simulink model "projet_working"  (R2018a)
settings: Solver=FixedStepAuto  StartTime=0.0  StopTime=5  RelTol=1e-3  EnableMultiTasking=on
values from neighbouring files (symbols this model uses):
  a = [0 1 ; 0 -6.523]    [Project_state_space.m]
  b = [0;1]    [Project_state_space.m]
  c = [0.09667 0]    [Project_state_space.m]
  k = place(sysssD.a,sysssD.b,[0.9 0.7])    [Discret_LEGO_script.m]    (also in Project_state_space.m = place(a, b, P'); RLS_Glemselsfaktor.m = Q*Phi'; RLS_Kalman.m = Q*Phi'; RLS_Online.m = p*Phi')
  L_1 = [l_1; l_2]    [Project_state_space.m]
libraries: legoev3lib x2
settings Model: SimulationMode=external  ExtModeTrigDuration=2  Creator=Lenovo  LastModifiedBy=Lenovo
settings SolverCC: PositivePriorityOrder=on
settings OptimizationCC: EnhancedBackFolding=on  PassReuseOutputArgsThreshold=0  MaxStackSize=64  OptimizeBlockOrder=speed  DifferentSizesBufferReuse=on  OptimizationCustomize=off
settings DebuggingCC: ParameterTunabilityLossMsg=error
settings HardwareCC: ProdBitPerPointer=32  ProdBitPerSizeT=32  ProdBitPerPtrDiffT=32  ProdLargestAtomicInteger=Long  ProdWordSize=32  ProdHWDeviceType=ARM Compatible->ARM 9  UseEmbeddedCoderFeatures=off  UseSimulinkCoderFeatures=off
settings SFSimCC: MATLABDynamicMemAlloc=off
settings RTWCC: SystemTargetFile=ert.tlc  HardwareBoard=LEGO MINDSTORMS EV3  TLCOptions="-aInlineSetEventsForThisBaseRateFcn=TLC_FALSE -aSuppressMultiTaskScheduler=TLC_FALSE  -aRateBasedStepFcn=0"  TemplateMakefile=ert_default_tmf  GenerateReport=on  Toolchain=Sourcery G++ Lite v2009q3  LaunchReport=on
settings CodeAppCC: ForceParamTrailComments=on  OperatorAnnotations=on
settings ERTTargetCC: ERTCustomFileBanners=off  SupportContinuousTime=on  SupportNonInlinedSFcns=on  RemoveResetFunc=off  SupportVariableSizeSignals=on  ModelStepFunctionPrototypeControlCompliant=off

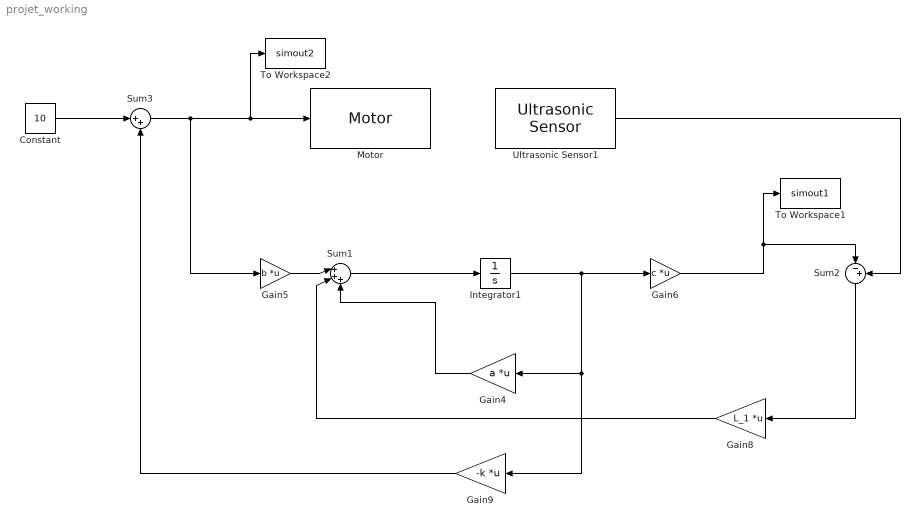
== system projet_working ==
  Constant : Constant  Value=10
  Gain4 : Gain  Gain=a  Multiplication=Matrix(K*u)
  Gain5 : Gain  Gain=b  Multiplication=Matrix(K*u)
  Gain6 : Gain  Gain=c  Multiplication=Matrix(K*u)
  Gain8 : Gain  Gain=L_1  Multiplication=Matrix(K*u)
  Gain9 : Gain  Gain=-k  Multiplication=Matrix(K*u)
  Integrator1 : Integrator
  Motor : legoev3lib/Motor  sportNumber=A  sstopAction=Brake
  Sum1 : Sum  Inputs=|+++
  Sum2 : Sum  Inputs=|-+
  Sum3 : Sum  Inputs=|++
  To Workspace1 : ToWorkspace  VariableName=simout1  SaveFormat=Structure With Time  SampleTime=-1
  To Workspace2 : ToWorkspace  VariableName=simout2  SaveFormat=Structure With Time  SampleTime=-1
  Ultrasonic Sensor1 : legoev3lib/Ultrasonic Sensor  PortNumber=1  sampleTime=0.1
      settings: SourceProductName=Simulink Support Package for LEGO MINDSTORMS EV3 Hardware  SourceProductBaseCode=LEGOEV3
  wires:
  Gain5/1 -> Sum1/1
  Gain9/1 -> Sum3/2
  Sum1/1 -> Integrator1/1
  Gain4/1 -> Sum1/3
  Sum2/1 -> Gain8/1
  Sum3/1 -> To Workspace2/1, Motor/1, Gain5/1
  Integrator1/1 -> Gain9/1, Gain4/1, Gain6/1
  Gain6/1 -> Sum2/1, To Workspace1/1
  Gain8/1 -> Sum1/2
  Ultrasonic Sensor1/1 -> Sum2/2
  Constant/1 -> Sum3/1
